simulink model "controller"  (R2024a)
settings: Solver=FixedStepAuto  StartTime=0.0  StopTime=10.0  FixedStep=1/100  RelTol=1e-3
undefined symbols (not defined in the file): MAX_TORQUE, MAX_TORQUE_REVERSE
settings Model: Creator=DAUIN-Win10  LastModifiedBy=lucap
settings OptimizationCC: ReuseModelBlockBuffer=off
settings DebuggingCC: UnconnectedInputMsg=warning  UnconnectedOutputMsg=warning  UnconnectedLineMsg=warning
settings ModelReferenceCC: EnableRefExpFcnMdlSchedulingChecks=on
settings RTWCC: GPUComputeCapability=3.5  DLArmComputeVersion=19.05

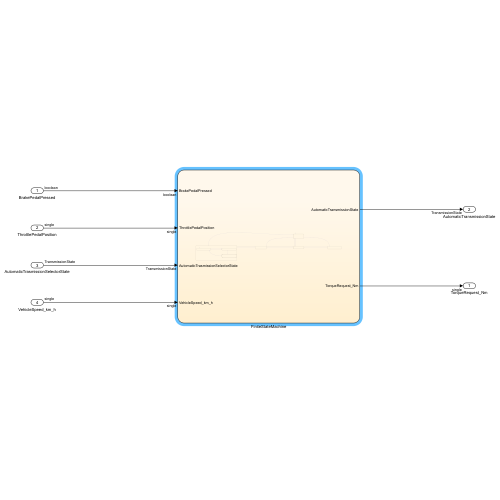
[thumbnail: Simulink's stored preview of the top-level diagram]
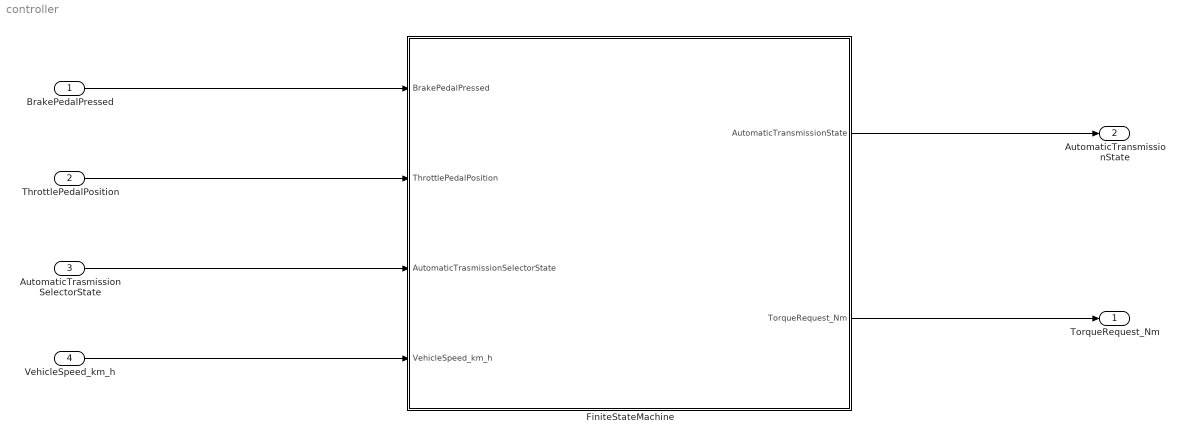
== system controller ==
  BrakePedalPressed : Inport  OutDataTypeStr=boolean
  ThrottlePedalPosition : Inport  Port=2  OutDataTypeStr=single
  AutomaticTrasmissionSelectorState : Inport  Port=3  OutDataTypeStr=Enum: TransmissionState
  VehicleSpeed_km_h : Inport  Port=4  OutDataTypeStr=single  Unit=km/h
  FiniteStateMachine : Stateflow chart  TreatAsAtomicUnit=on
  TorqueRequest_Nm : Outport  OutDataTypeStr=single  Unit=N*m
  AutomaticTransmissionState : Outport  Port=2  OutDataTypeStr=Enum: TransmissionState
  wires:
  BrakePedalPressed/1 -> FiniteStateMachine/1(BrakePedalPressed)
  ThrottlePedalPosition/1 -> FiniteStateMachine/2(ThrottlePedalPosition)
  AutomaticTrasmissionSelectorState/1 -> FiniteStateMachine/3(AutomaticTrasmissionSelectorState)
  VehicleSpeed_km_h/1 -> FiniteStateMachine/4(VehicleSpeed_km_h)
  FiniteStateMachine/1(AutomaticTransmissionState) -> AutomaticTransmissionState/1
  FiniteStateMachine/2(TorqueRequest_Nm) -> TorqueRequest_Nm/1

== stateflow chart controller/FiniteStateMachine ==
  state P
    entry:
    AutomaticTransmissionState = TransmissionState.Park
    TorqueRequest_Nm = 0
  state B
    entry:
    AutomaticTransmissionState = TransmissionState.Brake;
    state B_acc
      during:
      TorqueRequest_Nm = MAX_TORQUE * (3/2) * (ThrottlePedalPosition - 1/3)
    state B_dec
      during:
      TorqueRequest_Nm = -MAX_TORQUE * (1 - 3*ThrottlePedalPosition)
    state B_do_nothing
      entry:
      TorqueRequest_Nm = 0;
    B_acc -> B_dec : [ThrottlePedalPosition > 0 && ThrottlePedalPosition <= 1/3]
    B_dec -> B_acc [order 1] : [ThrottlePedalPosition > 1/3 && ThrottlePedalPosition <= 1]
    B_do_nothing -> B_acc : [ThrottlePedalPosition > 1/3 && ThrottlePedalPosition <= 1]
    B_dec -> B_do_nothing [order 2] : [VehicleSpeed_km_h <= 0]
    (default) -> B_do_nothing
  state D
    entry:
    AutomaticTransmissionState = TransmissionState.Drive
    during:
    TorqueRequest_Nm = MAX_TORQUE * ThrottlePedalPosition
  state N
    entry:
    AutomaticTransmissionState = TransmissionState.Neutral
    TorqueRequest_Nm = 0
  state R
    entry:
    AutomaticTransmissionState = TransmissionState.Reverse
    during:
    TorqueRequest_Nm = -MAX_TORQUE_REVERSE * ThrottlePedalPosition
  P -> B [order 2] : [ AutomaticTrasmissionSelectorState == TransmissionState.Brake && BrakePedalPressed == 1 && VehicleSpeed_km_h > -5]
  (default) -> P
  N -> P [order 2] : [abs(VehicleSpeed_km_h)<5 && BrakePedalPressed == 1 && AutomaticTrasmissionSelectorState == TransmissionState.Park]
  P -> N [order 1] : [AutomaticTrasmissionSelectorState == TransmissionState.Neutral && BrakePedalPressed == 1]
  B -> D : [AutomaticTrasmissionSelectorState == TransmissionState.Drive]
  D -> N [order 2] : [AutomaticTrasmissionSelectorState == TransmissionState.Neutral]
  N -> D [order 1] : [AutomaticTrasmissionSelectorState == TransmissionState.Drive && VehicleSpeed_km_h > -5 && BrakePedalPressed == 1]
  N -> R [order 3] : [VehicleSpeed_km_h < 5 && BrakePedalPressed == 1 && AutomaticTrasmissionSelectorState == TransmissionState.Reverse]
  D -> B [order 1] : [AutomaticTrasmissionSelectorState == TransmissionState.Brake]
  R -> N : [AutomaticTrasmissionSelectorState == TransmissionState.Neutral]
  data: BrakePedalPressed input; ThrottlePedalPosition input; AutomaticTrasmissionSelectorState input; VehicleSpeed_km_h input; AutomaticTransmissionState output; TorqueRequest_Nm output single; MAX_TORQUE parameter; MAX_TORQUE_REVERSE parameter
